simulink model "control_autonomous"  (R2012b)
settings: Solver=FixedStepDiscrete  StartTime=0.0  StopTime=300  RelTol=1e-3
values from neighbouring files (symbols this model uses):
  Kd = c2d(Krob,Ts)    [run_autonomous_control.m]
  Ts = 0.001    [run_autonomous_control.m]
undefined symbols (not defined in the file or in its folder): National_Instruments, PCI
libraries: rtwinlib x2, simulink x1
settings Model: SimulationMode=external  ExtModeTrigDuration=1000000  ExtModeArchiveMode=auto  ExtModeArchiveFileName=dataarch  ExtModeArchiveDirName=.\  Creator=f.cardoso-ribeiro  LastModifiedBy=f.cardoso-ribeiro
settings SolverCC: AutoInsertRateTranBlk=on
settings DataIOCC: LimitDataPoints=off  SaveOutput=off  SignalLogging=off  DSMLogging=off  SaveTime=off
settings HardwareCC: ProdIntDivRoundTo=Zero  ProdEndianess=LittleEndian  ProdHWDeviceType=Generic->32-bit x86 compatible
settings RTWCC: SystemTargetFile=rtwin.tlc  TemplateMakefile=rtwin.tmf  Description=Real-Time Windows Target  RTWVerbose=off  ProcessScript=rtwin_make_rtw_hook  RTWCompilerOptimization=On
settings CodeAppCC: MaxIdLength=95
settings RTWinTargetCC: TargetLibSuffix=_rtwin.lib  TargetPreCompLibLocation=C:\Program Files\MATLAB\R2012b\toolbox\rtw\targets\rtwin\lib\win64  CodeReplacementLibrary=ANSI_C  RTWinDir=C:/PROGRA~1/MATLAB/R2012b/toolbox/rtw/targets/rtwin  TargetArch=win64

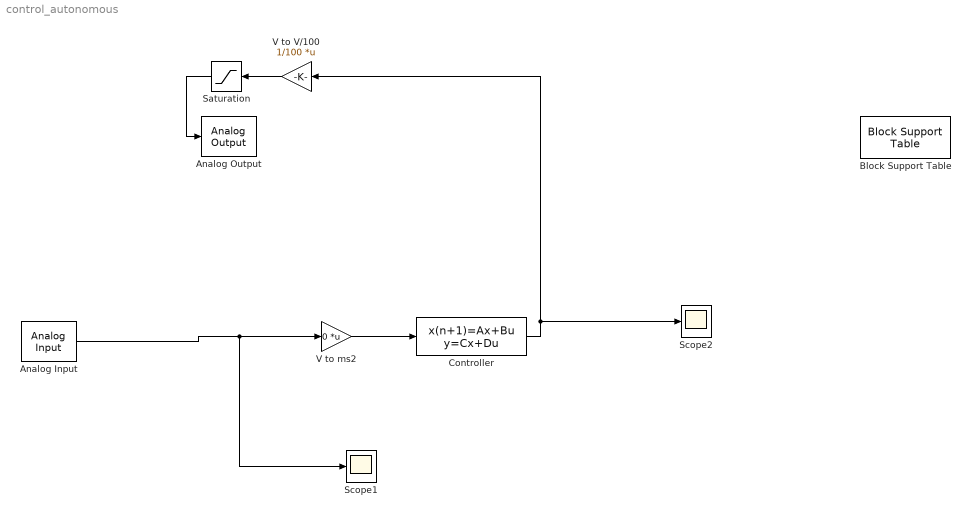
== system control_autonomous ==
  Analog Input : rtwinlib/Analog Input  SampleTime=0.0005  MaxMissedTicks=10  ShowMissedTicks=off  YieldWhenWaiting=off  DrvName=National_Instruments/PCI-6024E  DrvAddress=4294967295  DrvOptions=[1 0 0 0 0 0]  Channels=[1 2]  RangeMode=1  VoltRange=1  DataType=1
      settings: AttributesFormatString=National Instruments\nPCI-6024E [auto]
  Analog Output : rtwinlib/Analog Output  SampleTime=0.0005  MaxMissedTicks=10  ShowMissedTicks=off  YieldWhenWaiting=off  DrvName=National_Instruments/PCI-6024E  DrvAddress=4294967295  DrvOptions=[1 0 0 0 0 0]  Channels=[1 2]  RangeMode=1  VoltRange=1  InitialValue=0  FinalValue=0
      settings: AttributesFormatString=National Instruments\nPCI-6024E [auto]
  Block Support Table : simulink/Model-Wide Utilities/Block Support Table
  Controller : DiscreteStateSpace  A=Kd.A  B=Kd.B  C=Kd.C  D=Kd.D  SampleTime=Ts
  Saturation : Saturate  UpperLimit=1.5  LowerLimit=-1.5
  Scope1 : Scope
      settings: YMin=-0.35  YMax=0.35  SaveName=output
  Scope2 : Scope
      settings: YMin=-4  YMax=4.5  SaveName=input
  "V to V/100 " : Gain  Gain=1/100  Multiplication=Matrix(K*u)
  V to ms2 : Gain  Gain=0  Multiplication=Matrix(K*u)
  wires:
  Saturation/1 -> Analog Output/1
  Analog Input/1 -> Scope1/1, V to ms2/1
  "V to V/100 "/1 -> Saturation/1
  V to ms2/1 -> Controller/1
  Controller/1 -> "V to V/100 "/1, Scope2/1
